simulink model "FullCardioLablModel"  (R2023b)
settings: Solver=FixedStepDiscrete  StartTime=0.0  StopTime=param_sim_time  FixedStep=1/fs  MaxStep=1/fs  RelTol=1e-3
undefined symbols (not defined in the file): analyses, fdesignblkfcn, fs, gcbh, param_tot_samples
libraries: dspstat3 x13, SCGAnalysis_SignalGenerationLib x2
(part 19 of 20)

== matlab function FullCardioLablModel/SCG Analysis/Enabled SCG Analysis Subsystem/All Signals Signal Metric Characterization/SCG Systolic 3DMaxS1p2pProjection Signal Metric Characterization/Average Cycle-to-cycle Morphological Variability Calculator/Average Cycle-to-cycle Morphological Variability Calculator ==
  data: fs input size=[1]; r_pos input; scg_signal input; variability output size=[1]
function variability  = slk_morphological_variability_calculator(fs,r_pos,scg_signal)
% Simulink function to calculate an index of cycle-to-cycle morphological variability.

% INPUTS:
% r_pos = index positions of the R peaks of the ecg.
% scg_signal = signal to calculate its average cycle.

% OUTPUT:
% variability = cycle-to-cycle morphological variability.

% This function consists of three parts:
% Part 1 - Calculation of the (mean) average cycle.
% Part 2 - Calculation of the error signal of each cycle wrt to the average cycle.
% Part 3 - Calculation of rms value of the error signals of each cycle.
% Part 4 - Normalization of the rms value by dividing by (mean) average S1 p2p amplitude.


%% Part 1 - Calculation of the (mean) average cycle and the (mean) average S1 p2p amplitude.

% Calculating number of cycles to be considered in averaging (considered_cycles).
rr_min = min(diff(r_pos)); % Shortest cycle length - all the cycles will but cut down to this length.

if length(scg_signal) > r_pos(end) + rr_min
    considered_cycles = length(r_pos);
else
    considered_cycles = length(r_pos) - 1;
end

scg_signal_cycles = zeros(rr_min,considered_cycles); % Pre-initialization for speed.
s1p2pamp = zeros(considered_cycles,1);

% Isolating eafch cyle and calculating its S1 p2p amplitude.
for i = 1:considered_cycles
    scg_signal_cycles(:,i) = scg_signal(r_pos(i):r_pos(i) + rr_min - 1,1);
    s1p2pamp(i) = max(scg_signal_cycles(1:0.2*fs,i)) - min(scg_signal_cycles(1:0.2*fs,i)); % The S1 complex is considered as the 200ms following the detected R wave.
end

% Calculating the average cycle.
scg_signal_avg_cycle = mean(scg_signal_cycles,2);

% Calculating the average S1 p2p amplitude.
avg_s1p2pamp = mean(s1p2pamp);

rms_val = zeros(considered_cycles,1); % Pre-initialization for speed.
normalized_rms_val = zeros(considered_cycles,1);
variability = 0;

%% Part 2 - Calculation of the error signals.

error_signal = zeros(rr_min,considered_cycles); % Pre-initialization for speed.

for i = 1:considered_cycles
    error_signal(:,i) = scg_signal_cycles(:,i) - scg_signal_avg_cycle;
    
    %% Part 3 - Calculation of the rms values.
    rms_val(i) = rms(error_signal(:,i));
    
    %% Part 4 - Normalization of the rms values.
    normalized_rms_val(i) = rms_val(i)/avg_s1p2pamp;
end

variability = mean(normalized_rms_val,'all'); % The cycle-to-cycle morphological variability equals the mean normalized rms values of the error signals.

end

== matlab function FullCardioLablModel/SCG Analysis/Enabled SCG Analysis Subsystem/All Signals Signal Metric Characterization/SCG Systolic 3DMaxS1p2pProjection Signal Metric Characterization/Average S1 peak-to-peak Amplitude Calculator/Average S1p2p Amplitude Calculator ==
  data: fs input; r_pos input; scg_signal input; average_s1p2pamp output size=[1]
function average_s1p2pamp = slk_average_s1p2pamp_calculator(fs, r_pos, scg_signal)
% Function to calculate the average (mean) S1 peak-to-peak amplitude from an SCG input signal.

coder.extrinsic('sgtitle'); % Needed later for plotting.

num_cycles = length(r_pos);

s1p2pamp = zeros(1,num_cycles); % Pre-initialization for speed.
s1_peak_pos = zeros(1,num_cycles); 
s1_trough_pos = zeros(1,num_cycles); 
s1 = zeros(0.2*fs,1);

for i = 1:num_cycles 
    s1 = scg_signal(r_pos(i):r_pos(i) + 0.2*fs); % The S1 complex is considered as the 200ms following the R wave.
    s1_peak_pos(i) = r_pos(i) + find(s1 == max(s1));
    s1_trough_pos(i) = r_pos(i) + find(s1 == min(s1));
    s1p2pamp(i) = max(s1) - min(s1); % S1 peak-to-peak amplitude is the max minus the min inside the S1 window.   
end

average_s1p2pamp = mean(s1p2pamp);

%% Plotting.

figure;
sgtitle('SCG 3DMaxS1p2pProjection')
ax = [0 0]; % Pre-initialization

% Labelled SCG.
t = 0:1/fs:(length(scg_signal)-1)/fs;

ax(1) = subplot(2,1,1);
plot(t,scg_signal); hold on
plot((s1_peak_pos-1)/fs, scg_signal(s1_peak_pos), 'ro') % Plotting the peaks.
plot((s1_trough_pos-1)/fs, scg_signal(s1_trough_pos), 'bo') % Plotting the troughs.
ylim([min(scg_signal)-10 max(scg_signal)+10]);

% Green Vertical Lines to Denote R peak Positions.
for i = 1:num_cycles
    plot([(r_pos(i) - 1)/fs (r_pos(i) - 1)/fs],[min(scg_signal)-10 max(scg_signal)+10],'g--')
end

title('Labelled S1 Peaks + Troughs')
xlabel('Time (sec)')
ylabel('Acceleration (mg)')
box off

%% S1 p2p Amplitude Evolution.
ax(2) = subplot(2,1,2);
plot((((s1_peak_pos + s1_trough_pos)/2)-1)/fs, s1p2pamp,'.-'); hold on % Plotting the S1 P2P Amp. at the timepoints given by the midpoint between the detected S1 peaks and troughs.
xlabel('Time (sec)')
ylabel('Peak-to-Peak Amplitude (mg)')
title('S1 P2P Amplitude Evolution');
plot([0 (r_pos(end)-1)/fs], [average_s1p2pamp average_s1p2pamp],'r--') % Plotting the average S1 P2P Amp.
box off

linkaxes(ax,'x')

end

== matlab function FullCardioLablModel/SCG Analysis/Enabled SCG Analysis Subsystem/All Signals Signal Metric Characterization/SCG Systolic 3DMaxS1p2pProjection Signal Metric Characterization/Average S2 peak-to-peak Amplitude Calculator/Average S2p2p Amplitude Calculator ==
  data: fs input; r_pos input; scg_signal input; average_s2p2pamp output size=[1]
function average_s2p2pamp = slk_average_s2p2pamp_calculator(fs, r_pos, scg_signal)
% Function to calculate the average (mean) S2 peak-to-peak amplitude from an SCG input signal.

coder.extrinsic('sgtitle'); % Needed later for plotting.

num_cycles = length(r_pos);

s2p2pamp = zeros(1,num_cycles - 1); % Pre-initialization for speed.
s2_peak_pos = zeros(1,num_cycles - 1); 
s2_trough_pos = zeros(1,num_cycles - 1); 
s2_search_window_lims = [0.25*fs 0.5*fs]; % The window initially used to search for the S2 peak within that cycle.

for i = 1:num_cycles - 1 % The last heart cycle isn't considered because there's a signficant change that its S2 complex has been cut-off.
    
    cycle = scg_signal(r_pos(i):r_pos(i+1)); % The current heart cycle.
    
    s2_search_window = cycle(s2_search_window_lims(1):s2_search_window_lims(2)); % Defining the window where to search for the S2 peak.
    s2_peak_pos(i) = r_pos(i) + s2_search_window_lims(1) + find(s2_search_window==max(s2_search_window)); % Identifying the S2 peak.
    s2_trough_pos(i) = r_pos(i) + s2_search_window_lims(1) + find(s2_search_window==min(s2_search_window)); % Identifying the S2 trough.
    s2p2pamp(i)= scg_signal(s2_peak_pos(i)) - scg_signal(s2_trough_pos(i));
    
end

average_s2p2pamp = mean(s2p2pamp);

%% Plotting.

figure;
sgtitle('SCG 3DMaxS1p2pProjection')
ax = [0 0]; % Pre-initialization

% Labelled SCG.
t = 0:1/fs:(length(scg_signal)-1)/fs;

ax(1) = subplot(2,1,1);
plot(t,scg_signal); hold on
plot((s2_peak_pos-1)/fs, scg_signal(s2_peak_pos), 'ro') % Plotting the peaks.
plot((s2_trough_pos-1)/fs, scg_signal(s2_trough_pos), 'bo') % Plotting the troughs.
ylim([min(scg_signal)-10 max(scg_signal)+10]);

% Green Vertical Lines to Denote R peak Positions.
for i = 1:num_cycles
    plot([(r_pos(i) - 1)/fs (r_pos(i) - 1)/fs],[min(scg_signal)-10 max(scg_signal)+10],'g--')
end

title('Labelled S2 Peaks + Troughs')
xlabel('Time (sec)')
ylabel('Acceleration (mg)')
box off

%% S2 p2p Amplitude Evolution.
ax(2) = subplot(2,1,2);
plot((((s2_peak_pos + s2_trough_pos)/2) - 1)/fs, s2p2pamp,'.-'); hold on % Plotting the S2 P2P Amp. at the timepoints given by the midpoint between the detected S2 peaks and troughs.
xlabel('Time (sec)')
ylabel('Peak-to-Peak Amplitude (mg)')
title('S2 P2P Amplitude Evolution');
plot([0 (r_pos(end)-1)/fs], [average_s2p2pamp average_s2p2pamp],'r--') % Plotting the average S2 P2P Amp.
box off

linkaxes(ax,'x')

end

== matlab function FullCardioLablModel/SCG Analysis/Enabled SCG Analysis Subsystem/All Signals Signal Metric Characterization/SCG Systolic 3DMaxS1p2pProjection Signal Metric Characterization/Average Signal-to-Noise Ratio Calculator/Average S1 Signal-to-Noise Ratio/Average S1 SNR Calculator ==
  data: fs input size=[1]; r_pos input; scg_signal input; average_s1_snr output size=[1]
function average_s1_snr = slk_average_s1snr_calculator(fs, r_pos, scg_signal)
% Function to calculate the average (mean) S1 signal-to-noise ratio from an SCG input signal, where:
% Signal = S1 complex
% Noise = rest of cycle

% The signal-to-noise ratio is considered to be the ratio of
% root-mean-square values of the signal and the noise.

if r_pos
    
    num_cycles = length(r_pos);
    
    s1snr = zeros(1,num_cycles); % Pre-initialization for speed.
    
    for i = 1:num_cycles - 1
        signal = scg_signal(r_pos(i):r_pos(i) + 0.2*fs); % The signal is the S1 complex.
        noise = scg_signal(r_pos(i) + 0.2*fs + 1:r_pos(i+1)); % The rest of the cycle is the noise.
        s1snr(i) = rms(signal)/rms(noise); % SnR is the ratio of rms(signal) to rms (noise).
    end
    
    average_s1_snr = mean(s1snr);
    
else
    
    average_s1_snr = nan;
   
end

== matlab function FullCardioLablModel/SCG Analysis/Enabled SCG Analysis Subsystem/All Signals Signal Metric Characterization/SCG Systolic 3DMaxS1p2pProjection Signal Metric Characterization/Average Signal-to-Noise Ratio Calculator/Average S1X Signal-to-Noise Ratio/Average S1 SNR Amplitude Calculator ==
  data: fs input size=[1]; r_pos input; scg_signal input; average_s1x_snr output size=[1]
function average_s1x_snr = slk_average_s1xsnr_calculator(fs, r_pos, scg_signal)
% Function to calculate the average (mean) S1 signal-to-noise ratio from an SCG input signal, where:
% Signal = S1 complex
% Noise = rest of cycle EXCEPT the S2 complex

% The signal-to-noise ratio is considered to be the ratio of
% root-mean-square values of the signal and the noise.
    
num_cycles = length(r_pos);
s2_search_window_lims = [0.05*fs 0.3*fs]; % The window initially used to search for the S2 peak within the 'noise' segment.
s2_excise_window = fs*0.1; % The window length centered about the S2 peak (in samples) used to excise the S2 complex.

s1xsnr = zeros(1,num_cycles); % Pre-initialization for speed.

for i = 1:num_cycles - 1
    signal = scg_signal(r_pos(i):r_pos(i) + 0.2*fs); % The signal is the S1 complex.
 
    % Removing the S2 complex from the rest of the cycle.
    noise = scg_signal(1 + r_pos(i) + 0.2*fs:r_pos(i+1)); % Rest of the cycle.
    s2_search_window = noise(s2_search_window_lims(1):s2_search_window_lims(2)); % Defining the window where to search for the S2 peak.
    s2peak = s2_search_window_lims(1) + find(abs(s2_search_window) == max(abs(s2_search_window))); % Identifying the S2 peak within "noise".
    noise(s2peak(1) - s2_excise_window/2 : s2peak(1) + s2_excise_window/2) = []; % Removing the S2 complex.
    
    s1xsnr(i) = rms(signal)/rms(noise); % SnR is the ratio of rms(signal) to rms (noise).   
end

average_s1x_snr = mean(s1xsnr);

end

== matlab function FullCardioLablModel/SCG Analysis/Enabled SCG Analysis Subsystem/All Signals Signal Metric Characterization/SCG Systolic 3DMaxS1p2pProjection Signal Metric Characterization/Average Signal-to-Noise Ratio Calculator/Average S2 Signal-to-Noise Ratio/Average S2 SNR Calculator ==
  data: fs input size=[1]; r_pos input; scg_signal input; average_s2_snr output size=[1]
function average_s2_snr = slk_average_s2snr_calculator(fs, r_pos, scg_signal)
% Function to calculate the average (mean) S2 signal-to-noise ratio from an SCG input signal, where:
% Signal = S2 complex
% Noise = rest of cycle (including the S1 complex)

% The signal-to-noise ratio is considered to be the ratio of root-mean-square values of the signal and the noise.
    
num_cycles = length(r_pos);
s2_search_window_lims = [0.25*fs 0.5*fs]; % The window initially used to search for the S2 peak within that cycle.
s2_identify_window = fs*0.15; % The window length centered about the S2 peak (in samples) used to identify the S2 complex.

s2_snr = zeros(1,num_cycles); % Pre-initialization for speed.

for i = 1:num_cycles - 1 % The last cycle isn't considered because there's a good chance it's cut off.
   
    cycle = scg_signal(r_pos(i):r_pos(i+1)); % The current heart cycle.

    s2_search_window = cycle(s2_search_window_lims(1):s2_search_window_lims(2)); % Defining the window where to search for the S2 peak.
    s2peak = s2_search_window_lims(1) + find(abs(s2_search_window)==max(abs(s2_search_window))); % Identifying the S2 peak within 'cycle'.
    
    signal = cycle(s2peak(1) - s2_identify_window/2 : s2peak(1) + s2_identify_window/2); % The S2 complex is the signal.
    noise = cycle;
    noise(s2peak(1) - s2_identify_window/2 : s2peak(1) + s2_identify_window/2)= []; % Defining the noise as everything except the S2 complex.

    s2_snr(i) = rms(signal)/rms(noise);
    
end

average_s2_snr = mean(s2_snr);

end

== matlab function FullCardioLablModel/SCG Analysis/Enabled SCG Analysis Subsystem/All Signals Signal Metric Characterization/SCG Systolic 3DMaxS1p2pProjection Signal Metric Characterization/Average Signal-to-Noise Ratio Calculator/Average S2X Signal-to-Noise Ratio/Average S2X SNR Calculator ==
  data: fs input size=[1]; r_pos input; scg_signal input; average_s2x_snr output size=[1]
function average_s2x_snr = slk_average_s2xsnr_calculator(fs, r_pos, scg_signal)
% Function to calculate the average (mean) S2 signal-to-noise ratio from an SCG input signal, where:
% Signal = S2 complex
% Noise = rest of cycle EXCLUDING the S1 complex

% The signal-to-noise ratio is considered to be the ratio of root-mean-square values of the signal and the noise.
    
num_cycles = length(r_pos);
s1_excise_window_lims = [1 0.2*fs]; % The window used to excise the S1 complex from the noise.
s2_search_window_lims = [0.25*fs 0.5*fs]; % The window initially used to search for the S2 peak within that cycle.
s2_identify_window = fs*0.15; % The window length centered about the S2 peak (in samples) used to identify the S2 complex.

s2_snr = zeros(1,num_cycles); % Pre-initialization for speed.

for i = 1:num_cycles - 1
   
    cycle = scg_signal(r_pos(i):r_pos(i+1)); % The current heart cycle.

    s2_search_window = cycle(s2_search_window_lims(1):s2_search_window_lims(2)); % Defining the window where to search for the S2 peak.
    s2peak = s2_search_window_lims(1) + find(abs(s2_search_window) == max(abs(s2_search_window))); % Identifying the S2 peak within 'cycle'.
    
    signal = cycle(s2peak(1) - s2_identify_window/2 : s2peak(1) + s2_identify_window/2); % The S2 complex is the signal.
    noise = cycle;
    noise(s2peak(1) - s2_identify_window/2 : s2peak(1) + s2_identify_window/2)= []; % Removing the S2 complex from the noise.
    noise(s1_excise_window_lims(1):s1_excise_window_lims(2))= [];

    s2_snr(i) = rms(signal)/rms(noise);
    
end

average_s2x_snr = mean(s2_snr);

end

== matlab function FullCardioLablModel/SCG Analysis/Enabled SCG Analysis Subsystem/All Signals Signal Metric Characterization/SCG Systolic 3DMaxS1p2pProjection Signal Metric Characterization/Spectral Distribution Calculator/Spectral Distribution Calculator ==
  data: fs input size=[1]; r_pos input; scg_signal input; entire_cycle_nsd output size=[3 1]; entire_cycle_flag input size=[1]; s1_flag input size=[1]; s2_flag input size=[1]; f_band_lo input size=[1 2]; f_band_mid input size=[1 2]; f_band_hi input size=[1 2]; s1_nsd output size=[3 1]; s2_nsd output size=[3 1]
function [entire_cycle_nsd, s1_nsd, s2_nsd] = slk_normalized_spectral_distribution_calculator(fs, r_pos,scg_signal, entire_cycle_flag, s1_flag, s2_flag, f_band_lo, f_band_mid, f_band_hi)
% Simulink function to calculate the normalized spectral distribution of the power spectral densities of the entire cyle, the s1 complex, and the s2 complex, of an input SCG signal.

% INPUTS:
% fs = sampling frequency of scg_signal.
% r_pos = index positions of the R peaks of the ecg.
% scg_signal = signal to calculate its average cycle.
% entire_cycle_flag = flag to indicate the calculation of the entire cycle spectral distribution.
% s1_flag = flag to indicate the calculation of the S1 complex spectral distribution.
% s2_flag = flag to indicate the calculation of the S2 complex spectral distribution.

% OUTPUT:
% entire_cycle_nsd = normalized spectral distribution of the entire cycle (given as 3 elements corresponding to the spectral distribution in each of the 3 bins).
% s1_nsd = normalized spectral distribution of the s1 complex (given as 3 elements corresponding to the spectral distribution in each of the 3 bins).
% s2_nsd = normalized spectral distribution of the s2 complex (given as 3 elements corresponding to the spectral distribution in each of the 3 bins).

% This function consists of three parts:
% Part 1 - Calculation of the entire cycle normalized spectral distribution.
% Part 2 - Calculation of the S1 complex normalized spectral distribution.
% Part 3 - Calculation of the S2 complex normalized spectral distribution.

coder.extrinsic('legend');
coder.extrinsic('vline');

num_cycles = length(r_pos);

pad_size = 10*fs; % The length of the zero-padded vector used to obtain sufficient frequency resolution for the FFT.

PSDs = figure;
xlabel('Frequency (Hz)')
ylabel('Power Spectral Density (mg^2)')
xlim([0 f_band_hi(2)])
title('Power Spectral Densities')
hold on

freq_axis = fs*(0:pad_size/2)/pad_size; % Frequency axis for the FFT.

%% Part 1 - Calculation of the entire cycle normalized spectral distribution.


% if entire_cycle_flag
%     
%     current_cycle_padded = zeros(pad_size,1); % Pre-initializing for speed.
%     fft_entire_cycle_mag_2_sided = zeros(pad_size,1);
%     fft_entire_cycle_mag_1_sided = zeros(pad_size/2+1,num_cycles - 1);
%     
%     for i = 1:num_cycles - 1 % The last cycle isnt considered because it's not complete.
%         
%         current_cycle = scg_signal(r_pos(i):r_pos(i+1));
%         current_cycle_length = length(current_cycle); % In samples.
%         
%         % Ensuring the current cycle has an even number of samples - necessary for FFT calculation.
%         if mod(current_cycle_length,2) > 0
%             current_cycle_length = current_cycle_length - 1;
%             current_cycle(end) = [];
%         end
%                
%         current_cycle_padded = [current_cycle; zeros(pad_size - current_cycle_length,1)];
%         fft_entire_cycle = fft(current_cycle_padded); % (Complex) FFT values.
%         fft_entire_cycle_mag_2_sided = abs(fft_entire_cycle); % Two-sided Magnitude.
%         fft_entire_cycle_mag_1_sided(:,i) = fft_entire_cycle_mag_2_sided(1:length(current_cycle_padded)/2+1); % One-sided Magnitude.
%         fft_entire_cycle_mag_1_sided(2:end-1,i) = 2*fft_entire_cycle_mag_1_sided(2:end-1,i); % Multiplying by 2 to get total power (negative + positive frequencies).
%     end
%     
%     average_entire_cycle_fft = mean(fft_entire_cycle_mag_1_sided'); % The mean magnitude FFT spectrum.
%     
%     average_entire_cycle_psd = average_entire_cycle_fft.^2; % The power spectral density - the square of the magnitude spectrum.
%     
%     % Plotting.
%     figure(PSDs); hold on;
%     plot(freq_axis,average_entire_cycle_psd)
%     
%     % Integrating along the bands to get the bandpower.
%     entire_cycle_lo_power = trapz(ceil(f_band_lo(1)/freq_axis(2)):ceil(f_band_lo(2)/freq_axis(2)),average_entire_cycle_psd(ceil(f_band_lo(1)/freq_axis(2)):ceil(f_band_lo(2)/freq_axis(2))));
%     entire_cycle_mid_power = trapz(ceil(f_band_mid(1)/freq_axis(2)):ceil(f_band_mid(2)/freq_axis(2)),average_entire_cycle_psd(ceil(f_band_mid(1)/freq_axis(2)):ceil(f_band_mid(2)/freq_axis(2))));
%     entire_cycle_hi_power = trapz(ceil(f_band_hi(1)/freq_axis(2)):ceil(f_band_hi(2)/freq_axis(2)),average_entire_cycle_psd(ceil(f_band_hi(1)/freq_axis(2)):ceil(f_band_hi(2)/freq_axis(2))));
%     entire_cycle_total_power = trapz(ceil(f_band_lo(1)/freq_axis(2)):ceil(f_band_hi(2)/freq_axis(2)),average_entire_cycle_psd(ceil(f_band_lo(1)/freq_axis(2)):ceil(f_band_hi(2)/freq_axis(2))));
%     
%     % Dividing over total power to get the normalized spectral distribution (NSD).
%     normalized_entire_cycle_lo_power = entire_cycle_lo_power/entire_cycle_total_power;
%     normalized_entire_cycle_mid_power = entire_cycle_mid_power/entire_cycle_total_power;
%     normalized_entire_cycle_hi_power = entire_cycle_hi_power/entire_cycle_total_power;
%     
%     % Preparing outputs.
%     entire_cycle_nsd = [normalized_entire_cycle_lo_power;normalized_entire_cycle_mid_power;normalized_entire_cycle_hi_power];
%     
% else 
%     entire_cycle_nsd = [0; 0; 0];
% end


if entire_cycle_flag

    Interp_FFT_Cycle_Mag_1_Sided = zeros(num_cycles - 1, 10000); % Pre-initializing for speed.
    new_freq_axis_entire_cycle = linspace(0,fs/2,10000); % Interpolation frequency axis.

    for i = 1:num_cycles - 1 % The last cycle isnt considered because it's not complete.

        current_cycle = scg_signal(r_pos(i):r_pos(i+1));
        current_cycle_length = length(current_cycle); % In samples.

        % Ensuring the current cycle has an even number of samples - necessary for FFT calculation.
        if mod(current_cycle_length,2) > 0
            current_cycle_length = current_cycle_length - 1;
            current_cycle(end) = [];
        end

        FFT_Cycle = zeros(current_cycle_length,1); % Pre-initializing for speed.
        FFT_Cycle_Mag_2_Sided = zeros(current_cycle_length,1);
        FFT_Cycle_Mag_1_Sided = zeros(current_cycle_length/2+1,1);

        freq_axis_entire_cycle = fs*(0:current_cycle_length/2)/current_cycle_length; % Frequency axis for the FFT.

        % FFT of each individual cycle.
        FFT_Cycle = fft(current_cycle); % (Complex) FFT values.
        FFT_Cycle_Mag_2_Sided = abs(FFT_Cycle); % Two-sided Magnitude.
        FFT_Cycle_Mag_1_Sided = FFT_Cycle_Mag_2_Sided(1:current_cycle_length/2+1); % One-sided Magnitude.
        FFT_Cycle_Mag_1_Sided(2:end-1) = 2*FFT_Cycle_Mag_1_Sided(2:end-1); % Multiplying by 2 to get total power (negative + positive frequencies).

        % Interpolating to a new frequency axis. This is necessary because different cycles have different lenghts (and thus different FFT
        % lengths). To average the FFT across cycles, these must be interpolated to a particular fixed length.
        Interp_FFT_Cycle_Mag_1_Sided(i,:) = interp1(freq_axis_entire_cycle, FFT_Cycle_Mag_1_Sided, new_freq_axis_entire_cycle);

    end

    average_entire_cycle_FFT = mean(Interp_FFT_Cycle_Mag_1_Sided); % The mean magnitude FFT spectrum.

    average_entire_cycle_PSD = average_entire_cycle_FFT.^2; % The power spectral density - the square of the magnitude spectrum.

    % Plotting
    figure(PSDs);
    plot(new_freq_axis_entire_cycle,average_entire_cycle_PSD)

    % Integrating along the bands to get the bandpower.
    entire_cycle_lo_power = trapz(ceil(f_band_lo(1)/new_freq_axis_entire_cycle(2)):ceil(f_band_lo(2)/new_freq_axis_entire_cycle(2)),average_entire_cycle_PSD(ceil(f_band_lo(1)/new_freq_axis_entire_cycle(2)):ceil(f_band_lo(2)/new_freq_axis_entire_cycle(2))));
    entire_cycle_mid_power = trapz(ceil(f_band_mid(1)/new_freq_axis_entire_cycle(2)):ceil(f_band_mid(2)/new_freq_axis_entire_cycle(2)),average_entire_cycle_PSD(ceil(f_band_mid(1)/new_freq_axis_entire_cycle(2)):ceil(f_band_mid(2)/new_freq_axis_entire_cycle(2))));
    entire_cycle_hi_power = trapz(ceil(f_band_hi(1)/new_freq_axis_entire_cycle(2)):ceil(f_band_hi(2)/new_freq_axis_entire_cycle(2)),average_entire_cycle_PSD(ceil(f_band_hi(1)/new_freq_axis_entire_cycle(2)):ceil(f_band_hi(2)/new_freq_axis_entire_cycle(2))));
    entire_cycle_total_power = trapz(ceil(f_band_lo(1)/new_freq_axis_entire_cycle(2)):ceil(f_band_hi(2)/new_freq_axis_entire_cycle(2)),average_entire_cycle_PSD(ceil(f_band_lo(1)/new_freq_axis_entire_cycle(2)):ceil(f_band_hi(2)/new_freq_axis_entire_cycle(2))));

    % Dividing over total power to get the normalized spectral distribution (NSD).
    normalized_entire_cyce_lo_power = entire_cycle_lo_power/entire_cycle_total_power;
    normalized_entire_cyce_mid_power = entire_cycle_mid_power/entire_cycle_total_power;
    normalized_entire_cyce_hi_power = entire_cycle_hi_power/entire_cycle_total_power;

    % Preparing outputs.
    entire_cycle_nsd = [normalized_entire_cyce_lo_power;normalized_entire_cyce_mid_power;normalized_entire_cyce_hi_power];

    
else 
    entire_cycle_nsd = [0; 0; 0];

end

%% Part 2 - Calculation of the S1 complex normalized spectral distribution.

if s1_flag
    
    s1 = zeros(0.2*fs,1); % Pre-initializing for speed.
    s1_padded = zeros(pad_size,1);
    fft_s1_mag_2_sided = zeros(pad_size,1);
    fft_s1_mag_1_sided = zeros((pad_size)/2+1,num_cycles - 1);
    
    for i = 1:num_cycles - 1 % The last cycle isnt considered because there is a chance its S1 complex will be cut.
        s1 = scg_signal(r_pos(i):r_pos(i) + 0.2*fs - 1); % The S1 complex is considered as the 200ms following the ECG R peak.
        s1_padded = [s1; zeros(pad_size - 0.2*fs,1)];
        fft_s1 = fft(s1_padded); % (Complex) FFT values.
        fft_s1_mag_2_sided = abs(fft_s1); % Two-sided Magnitude.
        fft_s1_mag_1_sided(:,i) = fft_s1_mag_2_sided(1:length(s1_padded)/2+1); % One-sided Magnitude.
        fft_s1_mag_1_sided(2:end-1,i) = 2*fft_s1_mag_1_sided(2:end-1,i); % Multiplying by 2 to get total power (negative + positive frequencies).
    end
    
    average_s1_fft = mean(fft_s1_mag_1_sided'); % The mean magnitude FFT spectrum.
    
    average_s1_psd = average_s1_fft.^2; % The power spectral density - the square of the magnitude spectrum.
    
    % Plotting.
    figure(PSDs); hold on
    plot(freq_axis,average_s1_psd)
    
    % Integrating along the bands to get the bandpower.
    s1_lo_power = trapz(ceil(f_band_lo(1)/freq_axis(2)):ceil(f_band_lo(2)/freq_axis(2)),average_s1_psd(ceil(f_band_lo(1)/freq_axis(2)):ceil(f_band_lo(2)/freq_axis(2))));
    s1_mid_power = trapz(ceil(f_band_mid(1)/freq_axis(2)):ceil(f_band_mid(2)/freq_axis(2)),average_s1_psd(ceil(f_band_mid(1)/freq_axis(2)):ceil(f_band_mid(2)/freq_axis(2))));
    s1_hi_power = trapz(ceil(f_band_hi(1)/freq_axis(2)):ceil(f_band_hi(2)/freq_axis(2)),average_s1_psd(ceil(f_band_hi(1)/freq_axis(2)):ceil(f_band_hi(2)/freq_axis(2))));
    s1_total_power = trapz(ceil(f_band_lo(1)/freq_axis(2)):ceil(f_band_hi(2)/freq_axis(2)),average_s1_psd(ceil(f_band_lo(1)/freq_axis(2)):ceil(f_band_hi(2)/freq_axis(2))));
    
    % Dividing over total power to get the normalized spectral distribution (NSD).
    normalized_s1_lo_power = s1_lo_power/s1_total_power;
    normalized_s1_mid_power = s1_mid_power/s1_total_power;
    normalized_s1_hi_power = s1_hi_power/s1_total_power;
    
    % Preparing outputs.
    s1_nsd = [normalized_s1_lo_power;normalized_s1_mid_power;normalized_s1_hi_power];
    
else
    s1_nsd = [0; 0; 0;];
end

%% Part 3 - Calculation of the S2 complex normalized spectral distribution.

if s2_flag
    
    s2_search_window_lims = [0.25*fs 0.5*fs]; % The window initially used to search for the S2 peak within that cycle.
    s2_identify_window = 0.15*fs; % The window length centered about the S2 peak (in samples) used to identify the S2 complex.
    
    s2 = zeros(s2_identify_window,1); % Pre-initializing for speed.
    s2_padded = zeros(pad_size,1);
    fft_s2_mag_2_sided = zeros(pad_size,1);
    fft_s2_mag_1_sided = zeros((pad_size)/2+1,num_cycles - 1);
    
    for i = 1:num_cycles - 1 % The last cycle isnt considered because there is a chance its S1 complex will be cut.
        
        cycle = scg_signal(r_pos(i):r_pos(i+1)); % The current heart cycle.
        
        s2_search_window = cycle(s2_search_window_lims(1):s2_search_window_lims(2)); % Defining the window where to search for the S2 peak.
        s2peak = s2_search_window_lims(1) + find(abs(s2_search_window)==max(abs(s2_search_window))); % Identifying the S2 peak within 'cycle'.
        
        s2 = cycle(s2peak(1) - s2_identify_window/2 : s2peak(1) + s2_identify_window/2); % The S2 complex.
        s2_padded = [s2; zeros(pad_size - s2_identify_window - 1,1)]; % Padding the S2 complex with zeros.
        fft_s2 = fft(s2_padded); % (Complex) FFT values.
        fft_s2_mag_2_sided = abs(fft_s2); % Two-sided Magnitude.
        fft_s2_mag_1_sided(:,i) = fft_s2_mag_2_sided(1:length(s2_padded)/2+1); % One-sided Magnitude.
        fft_s2_mag_1_sided(2:end-1,i) = 2*fft_s2_mag_1_sided(2:end-1,i); % Multiplying by 2 to get total power (negative + positive frequencies).
    end
    
    average_s2_FFT = mean(fft_s2_mag_1_sided'); % The mean magnitude FFT spectrum.
    
    average_s2_PSD = average_s2_FFT.^2; % The power spectral density - the square of the magnitude spectrum.
    
    % Plotting.
    figure(PSDs); hold on;
    title('SCG 3D Systolic Max S1p2p Axis')
    plot(freq_axis,average_s2_PSD)
    
    % Integrating along the bands to get the bandpower.
    s2_lo_power = trapz(ceil(f_band_lo(1)/freq_axis(2)):ceil(f_band_lo(2)/freq_axis(2)),average_s2_PSD(ceil(f_band_lo(1)/freq_axis(2)):ceil(f_band_lo(2)/freq_axis(2))));
    s2_mid_power = trapz(ceil(f_band_mid(1)/freq_axis(2)):ceil(f_band_mid(2)/freq_axis(2)),average_s2_PSD(ceil(f_band_mid(1)/freq_axis(2)):ceil(f_band_mid(2)/freq_axis(2))));
    s2_hi_power = trapz(ceil(f_band_hi(1)/freq_axis(2)):ceil(f_band_hi(2)/freq_axis(2)),average_s2_PSD(ceil(f_band_hi(1)/freq_axis(2)):ceil(f_band_hi(2)/freq_axis(2))));
    s2_total_power = trapz(ceil(f_band_lo(1)/freq_axis(2)):ceil(f_band_hi(2)/freq_axis(2)),average_s2_PSD(ceil(f_band_lo(1)/freq_axis(2)):ceil(f_band_hi(2)/freq_axis(2))));
    
    % Dividing over total power to get the normalized spectral distribution (NSD).
    normalized_s2_lo_power = s2_lo_power/s2_total_power;
    normalized_s2_mid_power = s2_mid_power/s2_total_power;
    normalized_s2_hi_power = s2_hi_power/s2_total_power;
    
    % Preparing outputs.
    s2_nsd = [normalized_s2_lo_power;normalized_s2_mid_power;normalized_s2_hi_power];
    
else 
    s2_nsd = [0;0;0];    
end

% Plotting the frequency band delimiters
vline(f_band_lo(1),'r')
vline(f_band_mid(1),'r')
vline(f_band_hi(1),'r')
vline(f_band_hi(2),'r')

% Plotting the legend.
if entire_cycle_flag
    legend('Entire Cycle')
end

if s1_flag
    legend('S1')
end

if s2_flag
    legend('S2')
end

if entire_cycle_flag && s1_flag
    legend('Entire Cycle','S1')
end

if entire_cycle_flag && s2_flag
    legend('Entire Cycle','S2')
end

if s1_flag && s2_flag
    legend('S1','S2')
end

if entire_cycle_flag && s1_flag && s2_flag
    legend('Entire Cycle','S1','S2')
end

end

== matlab function FullCardioLablModel/SCG Analysis/Enabled SCG Analysis Subsystem/All Signals Signal Metric Characterization/SCG S2 3DAntiMechAxis Signal Metric Characterization/Average S1 peak-to-peak Amplitude Calculator/Average S1p2p Amplitude Calculator ==
  data: fs input; r_pos input; scg_signal input; average_s1p2pamp output size=[1]
function average_s1p2pamp = slk_average_s1p2pamp_calculator(fs, r_pos, scg_signal)
% Function to calculate the average (mean) S1 peak-to-peak amplitude from an SCG input signal.

coder.extrinsic('sgtitle'); % Needed later for plotting.

num_cycles = length(r_pos);

s1p2pamp = zeros(1,num_cycles); % Pre-initialization for speed.
s1_peak_pos = zeros(1,num_cycles); 
s1_trough_pos = zeros(1,num_cycles); 
s1 = zeros(0.2*fs,1);

for i = 1:num_cycles 
    s1 = scg_signal(r_pos(i):r_pos(i) + 0.2*fs); % The S1 complex is considered as the 200ms following the R wave.
    s1_peak_pos(i) = r_pos(i) + find(s1 == max(s1));
    s1_trough_pos(i) = r_pos(i) + find(s1 == min(s1));
    s1p2pamp(i) = max(s1) - min(s1); % S1 peak-to-peak amplitude is the max minus the min inside the S1 window.   
end

average_s1p2pamp = mean(s1p2pamp);

%% Plotting.

figure;
sgtitle('SCG S2 AntiMechAxis')
ax = [0 0]; % Pre-initialization

% Labelled SCG.
t = 0:1/fs:(length(scg_signal)-1)/fs;

ax(1) = subplot(2,1,1);
plot(t,scg_signal); hold on
plot((s1_peak_pos-1)/fs, scg_signal(s1_peak_pos), 'ro') % Plotting the peaks.
plot((s1_trough_pos-1)/fs, scg_signal(s1_trough_pos), 'bo') % Plotting the troughs.
ylim([min(scg_signal)-10 max(scg_signal)+10]);

% Green Vertical Lines to Denote R peak Positions.
for i = 1:num_cycles
    plot([(r_pos(i) - 1)/fs (r_pos(i) - 1)/fs],[min(scg_signal)-10 max(scg_signal)+10],'g--')
end

title('Labelled S1 Peaks + Troughs')
xlabel('Time (sec)')
ylabel('Acceleration (mg)')
box off

%% S1 p2p Amplitude Evolution.
ax(2) = subplot(2,1,2);
plot((((s1_peak_pos + s1_trough_pos)/2)-1)/fs, s1p2pamp,'.-'); hold on % Plotting the S1 P2P Amp. at the timepoints given by the midpoint between the detected S1 peaks and troughs.
xlabel('Time (sec)')
ylabel('Peak-to-Peak Amplitude (mg)')
title('S1 P2P Amplitude Evolution');
plot([0 (r_pos(end)-1)/fs], [average_s1p2pamp average_s1p2pamp],'r--') % Plotting the average S1 P2P Amp.
box off

linkaxes(ax,'x')

end

== matlab function FullCardioLablModel/SCG Analysis/Enabled SCG Analysis Subsystem/All Signals Signal Metric Characterization/SCG Systolic 3DMinS1p2pProjection Signal Metric Characterization/Average Cycle-to-cycle Morphological Variability Calculator/Average Cycle-to-cycle Morphological Variability Calculator ==
  data: fs input size=[1]; r_pos input; scg_signal input; variability output size=[1]
function variability  = slk_morphological_variability_calculator(fs,r_pos,scg_signal)
% Simulink function to calculate an index of cycle-to-cycle morphological variability.

% INPUTS:
% r_pos = index positions of the R peaks of the ecg.
% scg_signal = signal to calculate its average cycle.

% OUTPUT:
% variability = cycle-to-cycle morphological variability.

% This function consists of three parts:
% Part 1 - Calculation of the (mean) average cycle.
% Part 2 - Calculation of the error signal of each cycle wrt to the average cycle.
% Part 3 - Calculation of rms value of the error signals of each cycle.
% Part 4 - Normalization of the rms value by dividing by (mean) average S1 p2p amplitude.


%% Part 1 - Calculation of the (mean) average cycle and the (mean) average S1 p2p amplitude.

% Calculating number of cycles to be considered in averaging (considered_cycles).
rr_min = min(diff(r_pos)); % Shortest cycle length - all the cycles will but cut down to this length.

if length(scg_signal) > r_pos(end) + rr_min
    considered_cycles = length(r_pos);
else
    considered_cycles = length(r_pos) - 1;
end

scg_signal_cycles = zeros(rr_min,considered_cycles); % Pre-initialization for speed.
s1p2pamp = zeros(considered_cycles,1);

% Isolating eafch cyle and calculating its S1 p2p amplitude.
for i = 1:considered_cycles
    scg_signal_cycles(:,i) = scg_signal(r_pos(i):r_pos(i) + rr_min - 1,1);
    s1p2pamp(i) = max(scg_signal_cycles(1:0.2*fs,i)) - min(scg_signal_cycles(1:0.2*fs,i)); % The S1 complex is considered as the 200ms following the detected R wave.
end

% Calculating the average cycle.
scg_signal_avg_cycle = mean(scg_signal_cycles,2);

% Calculating the average S1 p2p amplitude.
avg_s1p2pamp = mean(s1p2pamp);

rms_val = zeros(considered_cycles,1); % Pre-initialization for speed.
normalized_rms_val = zeros(considered_cycles,1);
variability = 0;

%% Part 2 - Calculation of the error signals.

error_signal = zeros(rr_min,considered_cycles); % Pre-initialization for speed.

for i = 1:considered_cycles
    error_signal(:,i) = scg_signal_cycles(:,i) - scg_signal_avg_cycle;
    
    %% Part 3 - Calculation of the rms values.
    rms_val(i) = rms(error_signal(:,i));
    
    %% Part 4 - Normalization of the rms values.
    normalized_rms_val(i) = rms_val(i)/avg_s1p2pamp;
end

variability = mean(normalized_rms_val,'all'); % The cycle-to-cycle morphological variability equals the mean normalized rms values of the error signals.

end

== matlab function FullCardioLablModel/SCG Analysis/Enabled SCG Analysis Subsystem/All Signals Signal Metric Characterization/SCG Systolic 3DMinS1p2pProjection Signal Metric Characterization/Average S1 peak-to-peak Amplitude Calculator/Average S1p2p Amplitude Calculator ==
  data: fs input; r_pos input; scg_signal input; average_s1p2pamp output size=[1]
function average_s1p2pamp = slk_average_s1p2pamp_calculator(fs, r_pos, scg_signal)
% Function to calculate the average (mean) S1 peak-to-peak amplitude from an SCG input signal.

coder.extrinsic('sgtitle'); % Needed later for plotting.

num_cycles = length(r_pos);

s1p2pamp = zeros(1,num_cycles); % Pre-initialization for speed.
s1_peak_pos = zeros(1,num_cycles); 
s1_trough_pos = zeros(1,num_cycles); 
s1 = zeros(0.2*fs,1);

for i = 1:num_cycles 
    s1 = scg_signal(r_pos(i):r_pos(i) + 0.2*fs); % The S1 complex is considered as the 200ms following the R wave.
    s1_peak_pos(i) = r_pos(i) + find(s1 == max(s1));
    s1_trough_pos(i) = r_pos(i) + find(s1 == min(s1));
    s1p2pamp(i) = max(s1) - min(s1); % S1 peak-to-peak amplitude is the max minus the min inside the S1 window.   
end

average_s1p2pamp = mean(s1p2pamp);

%% Plotting.

figure;
sgtitle('SCG 3DMinS1p2pProjection')
ax = [0 0]; % Pre-initialization

% Labelled SCG.
t = 0:1/fs:(length(scg_signal)-1)/fs;

ax(1) = subplot(2,1,1);
plot(t,scg_signal); hold on
plot((s1_peak_pos-1)/fs, scg_signal(s1_peak_pos), 'ro') % Plotting the peaks.
plot((s1_trough_pos-1)/fs, scg_signal(s1_trough_pos), 'bo') % Plotting the troughs.
ylim([min(scg_signal)-10 max(scg_signal)+10]);

% Green Vertical Lines to Denote R peak Positions.
for i = 1:num_cycles
    plot([(r_pos(i) - 1)/fs (r_pos(i) - 1)/fs],[min(scg_signal)-10 max(scg_signal)+10],'g--')
end

title('Labelled S1 Peaks + Troughs')
xlabel('Time (sec)')
ylabel('Acceleration (mg)')
box off

%% S1 p2p Amplitude Evolution.
ax(2) = subplot(2,1,2);
plot((((s1_peak_pos + s1_trough_pos)/2)-1)/fs, s1p2pamp,'.-'); hold on % Plotting the S1 P2P Amp. at the timepoints given by the midpoint between the detected S1 peaks and troughs.
xlabel('Time (sec)')
ylabel('Peak-to-Peak Amplitude (mg)')
title('S1 P2P Amplitude Evolution');
plot([0 (r_pos(end)-1)/fs], [average_s1p2pamp average_s1p2pamp],'r--') % Plotting the average S1 P2P Amp.
box off

linkaxes(ax,'x')

end

== matlab function FullCardioLablModel/SCG Analysis/Enabled SCG Analysis Subsystem/All Signals Signal Metric Characterization/SCG Systolic 3DMinS1p2pProjection Signal Metric Characterization/Average S2 peak-to-peak Amplitude Calculator/Average S2p2p Amplitude Calculator ==
  data: fs input; r_pos input; scg_signal input; average_s2p2pamp output size=[1]
function average_s2p2pamp = slk_average_s2p2pamp_calculator(fs, r_pos, scg_signal)
% Function to calculate the average (mean) S2 peak-to-peak amplitude from an SCG input signal.

coder.extrinsic('sgtitle'); % Needed later for plotting.

num_cycles = length(r_pos);

s2p2pamp = zeros(1,num_cycles - 1); % Pre-initialization for speed.
s2_peak_pos = zeros(1,num_cycles - 1); 
s2_trough_pos = zeros(1,num_cycles - 1); 
s2_search_window_lims = [0.25*fs 0.5*fs]; % The window initially used to search for the S2 peak within that cycle.

for i = 1:num_cycles - 1 % The last heart cycle isn't considered because there's a signficant change that its S2 complex has been cut-off.
    
    cycle = scg_signal(r_pos(i):r_pos(i+1)); % The current heart cycle.
    
    s2_search_window = cycle(s2_search_window_lims(1):s2_search_window_lims(2)); % Defining the window where to search for the S2 peak.
    s2_peak_pos(i) = r_pos(i) + s2_search_window_lims(1) + find(s2_search_window==max(s2_search_window)); % Identifying the S2 peak.
    s2_trough_pos(i) = r_pos(i) + s2_search_window_lims(1) + find(s2_search_window==min(s2_search_window)); % Identifying the S2 trough.
    s2p2pamp(i)= scg_signal(s2_peak_pos(i)) - scg_signal(s2_trough_pos(i));
    
end

average_s2p2pamp = mean(s2p2pamp);

%% Plotting.

figure;
sgtitle('SCG 3DMinS1p2pProjection')
ax = [0 0]; % Pre-initialization

% Labelled SCG.
t = 0:1/fs:(length(scg_signal)-1)/fs;

ax(1) = subplot(2,1,1);
plot(t,scg_signal); hold on
plot((s2_peak_pos-1)/fs, scg_signal(s2_peak_pos), 'ro') % Plotting the peaks.
plot((s2_trough_pos-1)/fs, scg_signal(s2_trough_pos), 'bo') % Plotting the troughs.
ylim([min(scg_signal)-10 max(scg_signal)+10]);

% Green Vertical Lines to Denote R peak Positions.
for i = 1:num_cycles
    plot([(r_pos(i) - 1)/fs (r_pos(i) - 1)/fs],[min(scg_signal)-10 max(scg_signal)+10],'g--')
end

title('Labelled S2 Peaks + Troughs')
xlabel('Time (sec)')
ylabel('Acceleration (mg)')
box off

%% S2 p2p Amplitude Evolution.
ax(2) = subplot(2,1,2);
plot((((s2_peak_pos + s2_trough_pos)/2) - 1)/fs, s2p2pamp,'.-'); hold on % Plotting the S2 P2P Amp. at the timepoints given by the midpoint between the detected S2 peaks and troughs.
xlabel('Time (sec)')
ylabel('Peak-to-Peak Amplitude (mg)')
title('S2 P2P Amplitude Evolution');
plot([0 (r_pos(end)-1)/fs], [average_s2p2pamp average_s2p2pamp],'r--') % Plotting the average S2 P2P Amp.
box off

linkaxes(ax,'x')

end

== matlab function FullCardioLablModel/SCG Analysis/Enabled SCG Analysis Subsystem/All Signals Signal Metric Characterization/SCG Systolic 3DMinS1p2pProjection Signal Metric Characterization/Average Signal-to-Noise Ratio Calculator/Average S1 Signal-to-Noise Ratio/Average S1 SNR Calculator ==
  data: fs input size=[1]; r_pos input; scg_signal input; average_s1_snr output size=[1]
function average_s1_snr = slk_average_s1snr_calculator(fs, r_pos, scg_signal)
% Function to calculate the average (mean) S1 signal-to-noise ratio from an SCG input signal, where:
% Signal = S1 complex
% Noise = rest of cycle

% The signal-to-noise ratio is considered to be the ratio of
% root-mean-square values of the signal and the noise.

if r_pos
    
    num_cycles = length(r_pos);
    
    s1snr = zeros(1,num_cycles); % Pre-initialization for speed.
    
    for i = 1:num_cycles - 1
        signal = scg_signal(r_pos(i):r_pos(i) + 0.2*fs); % The signal is the S1 complex.
        noise = scg_signal(r_pos(i) + 0.2*fs + 1:r_pos(i+1)); % The rest of the cycle is the noise.
        s1snr(i) = rms(signal)/rms(noise); % SnR is the ratio of rms(signal) to rms (noise).
    end
    
    average_s1_snr = mean(s1snr);
    
else
    
    average_s1_snr = nan;
   
end

== matlab function FullCardioLablModel/SCG Analysis/Enabled SCG Analysis Subsystem/All Signals Signal Metric Characterization/SCG Systolic 3DMinS1p2pProjection Signal Metric Characterization/Average Signal-to-Noise Ratio Calculator/Average S1X Signal-to-Noise Ratio/Average S1 SNR Amplitude Calculator ==
  data: fs input size=[1]; r_pos input; scg_signal input; average_s1x_snr output size=[1]
function average_s1x_snr = slk_average_s1xsnr_calculator(fs, r_pos, scg_signal)
% Function to calculate the average (mean) S1 signal-to-noise ratio from an SCG input signal, where:
% Signal = S1 complex
% Noise = rest of cycle EXCEPT the S2 complex

% The signal-to-noise ratio is considered to be the ratio of
% root-mean-square values of the signal and the noise.
    
num_cycles = length(r_pos);
s2_search_window_lims = [0.05*fs 0.3*fs]; % The window initially used to search for the S2 peak within the 'noise' segment.
s2_excise_window = fs*0.1; % The window length centered about the S2 peak (in samples) used to excise the S2 complex.

s1xsnr = zeros(1,num_cycles); % Pre-initialization for speed.

for i = 1:num_cycles - 1
    signal = scg_signal(r_pos(i):r_pos(i) + 0.2*fs); % The signal is the S1 complex.
 
    % Removing the S2 complex from the rest of the cycle.
    noise = scg_signal(1 + r_pos(i) + 0.2*fs:r_pos(i+1)); % Rest of the cycle.
    s2_search_window = noise(s2_search_window_lims(1):s2_search_window_lims(2)); % Defining the window where to search for the S2 peak.
    s2peak = s2_search_window_lims(1) + find(abs(s2_search_window) == max(abs(s2_search_window))); % Identifying the S2 peak within "noise".
    noise(s2peak(1) - s2_excise_window/2 : s2peak(1) + s2_excise_window/2) = []; % Removing the S2 complex.
    
    s1xsnr(i) = rms(signal)/rms(noise); % SnR is the ratio of rms(signal) to rms (noise).   
end

average_s1x_snr = mean(s1xsnr);

end

== matlab function FullCardioLablModel/SCG Analysis/Enabled SCG Analysis Subsystem/All Signals Signal Metric Characterization/SCG Systolic 3DMinS1p2pProjection Signal Metric Characterization/Average Signal-to-Noise Ratio Calculator/Average S2 Signal-to-Noise Ratio/Average S2 SNR Calculator ==
  data: fs input size=[1]; r_pos input; scg_signal input; average_s2_snr output size=[1]
function average_s2_snr = slk_average_s2snr_calculator(fs, r_pos, scg_signal)
% Function to calculate the average (mean) S2 signal-to-noise ratio from an SCG input signal, where:
% Signal = S2 complex
% Noise = rest of cycle (including the S1 complex)

% The signal-to-noise ratio is considered to be the ratio of root-mean-square values of the signal and the noise.
    
num_cycles = length(r_pos);
s2_search_window_lims = [0.25*fs 0.5*fs]; % The window initially used to search for the S2 peak within that cycle.
s2_identify_window = fs*0.15; % The window length centered about the S2 peak (in samples) used to identify the S2 complex.

s2_snr = zeros(1,num_cycles); % Pre-initialization for speed.

for i = 1:num_cycles - 1 % The last cycle isn't considered because there's a good chance it's cut off.
   
    cycle = scg_signal(r_pos(i):r_pos(i+1)); % The current heart cycle.

    s2_search_window = cycle(s2_search_window_lims(1):s2_search_window_lims(2)); % Defining the window where to search for the S2 peak.
    s2peak = s2_search_window_lims(1) + find(abs(s2_search_window)==max(abs(s2_search_window))); % Identifying the S2 peak within 'cycle'.
    
    signal = cycle(s2peak(1) - s2_identify_window/2 : s2peak(1) + s2_identify_window/2); % The S2 complex is the signal.
    noise = cycle;
    noise(s2peak(1) - s2_identify_window/2 : s2peak(1) + s2_identify_window/2)= []; % Defining the noise as everything except the S2 complex.

    s2_snr(i) = rms(signal)/rms(noise);
    
end

average_s2_snr = mean(s2_snr);

end

== matlab function FullCardioLablModel/SCG Analysis/Enabled SCG Analysis Subsystem/All Signals Signal Metric Characterization/SCG Systolic 3DMinS1p2pProjection Signal Metric Characterization/Average Signal-to-Noise Ratio Calculator/Average S2X Signal-to-Noise Ratio/Average S2X SNR Calculator ==
  data: fs input size=[1]; r_pos input; scg_signal input; average_s2x_snr output size=[1]
function average_s2x_snr = slk_average_s2xsnr_calculator(fs, r_pos, scg_signal)
% Function to calculate the average (mean) S2 signal-to-noise ratio from an SCG input signal, where:
% Signal = S2 complex
% Noise = rest of cycle EXCLUDING the S1 complex

% The signal-to-noise ratio is considered to be the ratio of root-mean-square values of the signal and the noise.
    
num_cycles = length(r_pos);
s1_excise_window_lims = [1 0.2*fs]; % The window used to excise the S1 complex from the noise.
s2_search_window_lims = [0.25*fs 0.5*fs]; % The window initially used to search for the S2 peak within that cycle.
s2_identify_window = fs*0.15; % The window length centered about the S2 peak (in samples) used to identify the S2 complex.

s2_snr = zeros(1,num_cycles); % Pre-initialization for speed.

for i = 1:num_cycles - 1
   
    cycle = scg_signal(r_pos(i):r_pos(i+1)); % The current heart cycle.

    s2_search_window = cycle(s2_search_window_lims(1):s2_search_window_lims(2)); % Defining the window where to search for the S2 peak.
    s2peak = s2_search_window_lims(1) + find(abs(s2_search_window) == max(abs(s2_search_window))); % Identifying the S2 peak within 'cycle'.
    
    signal = cycle(s2peak(1) - s2_identify_window/2 : s2peak(1) + s2_identify_window/2); % The S2 complex is the signal.
    noise = cycle;
    noise(s2peak(1) - s2_identify_window/2 : s2peak(1) + s2_identify_window/2)= []; % Removing the S2 complex from the noise.
    noise(s1_excise_window_lims(1):s1_excise_window_lims(2))= [];

    s2_snr(i) = rms(signal)/rms(noise);
    
end

average_s2x_snr = mean(s2_snr);

end
